simulink library "GTMLE_Library"  (R2014a)
settings: Solver=ode45  StartTime=0.0  StopTime=10.0  RelTol=1e-3
undefined symbols (not defined in the file or in its folder): CCP, DiscIntNeverNeededParam, DPos_test, sample_time, TData_test
undefined symbols (not defined in the file): MCP, steadydata
libraries: simulink x10, GTMLE_Library x2, discretizing x1
(part 2 of 2)

== system GTMLE_Library/Control/Static Control/ /Kp_cor to Kp ==
  Kp_cor : Inport
  T2 : Inport  Port=2
  Fcn : Fcn  Expr=u(1)*sqrt(u(2)/288.15)
  Mux : Mux  Inputs=2
  Kp : Outport
  wires:
  Mux/1 -> Fcn/1
  T2/1 -> Mux/2
  Fcn/1 -> Kp/1
  Kp_cor/1 -> Mux/1

== system GTMLE_Library/Control/Static Control/ /N1_cor ==
  N1 : Inport
  T2 : Inport  Port=2
  Fcn : Fcn  Expr=(u(1)/sqrt(u(2)))*sqrt(288.15)
  Mux : Mux  Inputs=2
  N1cor : Outport
  wires:
  N1/1 -> Mux/1
  Mux/1 -> Fcn/1
  Fcn/1 -> N1cor/1
  T2/1 -> Mux/2

== system GTMLE_Library/Effectors/Iterative NR Solver w JacobianCalc/JC w Reset/Jacobian Calculator ==
  Reset : Inport
  f(x_p) : Inport  Port=2
  Xo : Inport  Port=3
  Constant2 : Constant  Value=N_Per_M
  Counter : Subsystem  mask{N_Ind_M=length(N_Per_M)}
      mask prompts: N_Ind_M "number of independents, N_Ind_M"
  Jacobian : Subsystem
  Terminator : Terminator
  J : Outport
  x_p : Outport  Port=2
  Iteration : Outport  Port=3
  Active : Outport  Port=4
  inv(J) : Outport  Port=5
  wires:
  f(x_p)/1 -> Jacobian/3(f(x_p))
  Constant2/1 -> Jacobian/2(Per)
  Jacobian/1(x_p) -> x_p/1
  Reset/1 -> Counter/1(Reset)
  Counter/1(Enable) -> Active/1, Jacobian/Enable
  Xo/1 -> Jacobian/4(Xo)
  Counter/2(Iteration) -> Iteration/1, Jacobian/1(Iteration)
  Jacobian/2(Inv(J)) -> inv(J)/1
  Jacobian/3(J) -> J/1
  Jacobian/4(y_State) -> Terminator/1

== system GTMLE_Library/Effectors/Iterative NR Solver w JacobianCalc/NRwCond/Iteration Conditions ==
  f(x) : Inport
  Abs : Abs
  Constant1 : Constant  Value=Cond_Limits_M
  Constant2 : Constant  Value=0
  Relational Operator : RelationalOperator  Operator=>  OutDataTypeStr=boolean
  Relational Operator1 : RelationalOperator  Operator=>  OutDataTypeStr=boolean
  Sum of Elements : Sum  Inputs=+
  Condition : Outport
  wires:
  Relational Operator1/1 -> Condition/1
  Sum of Elements/1 -> Relational Operator1/1
  Constant2/1 -> Relational Operator1/2
  Relational Operator/1 -> Sum of Elements/1
  f(x)/1 -> Abs/1
  Constant1/1 -> Relational Operator/2
  Abs/1 -> Relational Operator/1

== system GTMLE_Library/Effectors/Iterative NR Solver w JacobianCalc/NRwCond/Newton Raphson Solver ==
  Enable : Inport
  inv(f'(x(n))) : Inport  Port=2
  f(x(n)) : Inport  Port=3
  Data Type Conversion : DataTypeConversion
  MatrixMult : Subsystem
  Product1 : Product  RndMeth=Zero
  Product2 : Product  RndMeth=Zero
  Sum : Sum  Inputs=|-+
  Unit Delay : UnitDelay  InitialCondition=NR_IC_M  SampleTime=-1
  dxLimit : Subsystem
  x(n+1) : Outport
  y(n) : Outport  Port=2
  wires:
  inv(f'(x(n)))/1 -> Product2/1
  f(x(n))/1 -> Product1/1
  MatrixMult/1(DTS) -> dxLimit/1(dx)
  dxLimit/1(dx_limited) -> Sum/1
  Sum/1 -> y(n)/1, Unit Delay/1
  Unit Delay/1 -> Sum/2, dxLimit/2(dx1), x(n+1)/1
  Product1/1 -> MatrixMult/1(f(x(n)))
  Product2/1 -> MatrixMult/2(inv(f'(x(n))))
  Enable/1 -> Data Type Conversion/1
  Data Type Conversion/1 -> Product1/2, Product2/2

== system GTMLE_Library/Effectors/Iterative NR Solver w JacobianCalc/JC w Reset/Jacobian Calculator/Counter ==
  Reset : Inport
  Constant : Constant
  Constant1 : Constant  Value=N_Ind_M
  Constant2 : Constant  Value=3
  Logical Operator1 : Logic  Operator=NOT  AllPortsSameDT=off  OutDataTypeStr=boolean
  MinMax1 : MinMax  Inputs=2
  Product : Product  RndMeth=Zero
  Relational Operator : RelationalOperator  Operator=>  OutDataTypeStr=boolean
  Sum : Sum  Inputs=|++
  Sum1 : Sum  Inputs=|++
  Unit Delay : UnitDelay  SampleTime=-1
  Enable : Outport
  Iteration : Outport  Port=2
  wires:
  Constant/1 -> Sum/1
  Product/1 -> MinMax1/1
  Sum/1 -> MinMax1/2
  Unit Delay/1 -> Sum/2
  MinMax1/1 -> Unit Delay/1, Iteration/1, Relational Operator/2
  Relational Operator/1 -> Enable/1
  Logical Operator1/1 -> Product/2
  Reset/1 -> Logical Operator1/1
  Sum1/1 -> Relational Operator/1, Product/1
  Constant2/1 -> Sum1/2
  Constant1/1 -> Sum1/1

== system GTMLE_Library/Effectors/Iterative NR Solver w JacobianCalc/JC w Reset/Jacobian Calculator/Jacobian ==
  Iteration : Inport
  Per : Inport  Port=2
  f(x_p) : Inport  Port=3
  Xo : Inport  Port=4
  Enable : EnablePort
  Jacobian Calc : MATLAB Function  TreatAsAtomicUnit=on
  Unit Delay : UnitDelay  InitialCondition=zeros(length(N_Per_M),length(N_Per_M))  SampleTime=-1
  Unit Delay1 : UnitDelay  InitialCondition=zeros(length(N_Per_M),length(N_Per_M)+1)  SampleTime=-1
  Unit Delay2 : UnitDelay  InitialCondition=zeros(length(N_Per_M),1)  SampleTime=-1
  x_p : Outport
  Inv(J) : Outport  Port=2
  J : Outport  Port=3
  y_State : Outport  Port=4
  wires:
  Jacobian Calc/1(XpOut) -> x_p/1
  Xo/1 -> Jacobian Calc/4(XoIn)
  Per/1 -> Jacobian Calc/3(PerIn)
  Iteration/1 -> Jacobian Calc/1(IterationIn)
  Jacobian Calc/3(JOut) -> Unit Delay/1, J/1
  Jacobian Calc/2(InvJOut) -> Inv(J)/1
  Unit Delay/1 -> Jacobian Calc/5(JStateIn)
  Jacobian Calc/4(y_StateOut) -> y_State/1, Unit Delay1/1
  Unit Delay1/1 -> Jacobian Calc/6(y_StateIn)
  f(x_p)/1 -> Unit Delay2/1
  Unit Delay2/1 -> Jacobian Calc/2(y_xpIn)

== system GTMLE_Library/Effectors/Iterative NR Solver w JacobianCalc/NRwCond/Newton Raphson Solver/MatrixMult ==
  f(x(n)) : Inport
  inv(f'(x(n))) : Inport  Port=2
  Product : Product  Multiplication=Matrix(*)  RndMeth=Zero
  DTS : Outport
  wires:
  Product/1 -> DTS/1
  f(x(n))/1 -> Product/2
  inv(f'(x(n)))/1 -> Product/1

== system GTMLE_Library/Effectors/Iterative NR Solver w JacobianCalc/NRwCond/Newton Raphson Solver/dxLimit ==
  dx : Inport
  dx1 : Inport  Port=2
  Abs : Abs
  Constant : Constant  Value=0.5
  Constant1 : Constant  Value=-1
  MinMax : MinMax  Inputs=2
  MinMax1 : MinMax  Function=max  Inputs=2
  Product1 : Product  Inputs=3  RndMeth=Zero
  Product2 : Product  RndMeth=Zero
  Sum : Sum  Inputs=|++
  Threshold : Constant  Value=NR_dx_Lim_M/100
  Unit Delay : UnitDelay  InitialCondition=NR_IC_M  SampleTime=-1
  dx_limited : Outport
  wires:
  MinMax1/1 -> dx_limited/1
  Constant1/1 -> Product2/1
  Product2/1 -> MinMax1/1
  MinMax/1 -> MinMax1/2
  dx/1 -> MinMax/2
  Abs/1 -> Product2/2, MinMax/1
  Product1/1 -> Abs/1
  Threshold/1 -> Product1/1
  dx1/1 -> Sum/2, Unit Delay/1
  Constant/1 -> Product1/2
  Unit Delay/1 -> Sum/1
  Sum/1 -> Product1/3

== matlab function GTMLE_Library/Turbo/Compressor/Comp ==
  data: GasPthCharIn input; GasPthCharOut output; PwrOut output; NErrorOut output; OthrData output; CustBldsCharOut output size=[5 size(CustBldsPlan,2)]; FBldsCharOut output size=[5 size(FBldsPlan,2)]; Nmech input; beta_guess input; VSV input; CustBldsPlan input; FBldsPlan input; Nc_tab input; Beta_tab input; Eff_tab input; PR_tab input; Wc_tab input; SF input; CNST input; WcSurgeVec input; PRSurgeVec input; Msg output
function [ GasPthCharOut, PwrOut, NErrorOut, OthrData, CustBldsCharOut, FBldsCharOut, Msg ] = ComponentsComp( GasPthCharIn, Nmech, beta_guess, VSV, CustBldsPlan, FBldsPlan, Nc_tab, Beta_tab, Eff_tab, PR_tab, Wc_tab, SF, CNST, WcSurgeVec, PRSurgeVec )

[ GasPthCharOut, PwrOut, NErrorOut, OthrData, CustBldsCharOut, FBldsCharOut, Msg ] = Compressor_Untitled( GasPthCharIn, Nmech, beta_guess, VSV, CustBldsPlan, FBldsPlan, Nc_tab, Beta_tab, Eff_tab, PR_tab, Wc_tab, SF, CNST, WcSurgeVec, PRSurgeVec );

end

== matlab function GTMLE_Library/Turbo/Turbine/Turb ==
  data: CoolingFlwCharIn input; GasPthCharIn input size=[5 1]; GasPthCharOut output size=[5 1]; PwrOut output; NErrorOut output; OthrData output; Nmech input; PR input; CoolingPlan input; Nc_tab input; Eff_tab input; PR_tab input; Wc_tab input; SF input; CNST input; Msg output; FuelType input
function [ GasPthCharOut, PwrOut, NErrorOut, OthrData, Msg ] = ComponentsTurb( CoolingFlwCharIn, GasPthCharIn, Nmech, PR, CoolingPlan, Nc_tab, Eff_tab, PR_tab, Wc_tab, SF, CNST, FuelType )

[ GasPthCharOut, PwrOut, NErrorOut, OthrData, Msg ] = Turbine_Untitled( CoolingFlwCharIn, GasPthCharIn, Nmech, PR, CoolingPlan, Nc_tab, Eff_tab, PR_tab, Wc_tab, SF, CNST, FuelType );
   
end

== matlab function GTMLE_Library/Turbo/Duct/Duct ==
  data: GasPthCharIn input size=[5 1]; GasPthCharOut output; CNST input; PtIn_des input; TtIn_des input; WIn_des input; sigma_des input; Blds input; OthrData output
function [ GasPthCharOut, OthrData ]  = ComponentsDuct ( GasPthCharIn , CNST, PtIn_des, TtIn_des, WIn_des, sigma_des, Blds )

[ GasPthCharOut, OthrData ] = Duct_Untitled ( GasPthCharIn , CNST, PtIn_des, TtIn_des, WIn_des, sigma_des, Blds );

end

== matlab function GTMLE_Library/Effectors/Mixer_Ades_calc/MATLAB Function ==
  data: GasPthCharIn1 input; Ades1 output; GasPthCharIn2 input; Mades1 input; Mades2 input; Ades2 output
%%%%%%%%%%%%%%%%%%%%%%%%%%%%%%%%%%
% Untitled -- Mixer_Ades_calc_Untitled.c
% written by Miao Keqiang
% Aeroengine Control Library, Beihang University
% July 12th, 2015

% version 1.0

%%%%%%%%%%%%%%%%%%%%%%%%%%%%%%%%%%

function [ Ades1, Ades2 ] = Mixer_Ades_cal( GasPthCharIn1, GasPthCharIn2, Mades1, Mades2 )

% -- Load data --

WIn1 = 0;
TtIn1 = 0;
PtIn1 = 0;
FARcIn1 = 0;
WIn2 = 0;
TtIn2 = 0;
PtIn2 = 0;
FARcIn2 = 0;

if length( GasPthCharIn1 ) == 5
WIn1 = GasPthCharIn1( 1 );
TtIn1 = GasPthCharIn1( 3 );
PtIn1 = GasPthCharIn1( 4 );
FARcIn1 = GasPthCharIn1( 5 );
end

if length( GasPthCharIn2 ) == 5
WIn2 = GasPthCharIn2( 1 );
TtIn2 = GasPthCharIn2( 3 );
PtIn2 = GasPthCharIn2( 4 );
FARcIn2 = GasPthCharIn2( 5 );
end


% --  Calculate Kq & qlambda1 --

RIn1 = gas_constant( FARcIn1 );
CpIn1 = Cp_T( TtIn1, FARcIn1 );
gammaIn1 = CpIn1 / (CpIn1 - RIn1);
Kqlambda1 = sqrt( gammaIn1/RIn1*( (2/(gammaIn1+1))^((gammaIn1+1)/(gammaIn1-1)) ) );
lambda1 = sqrt( (gammaIn1 + 1) / 2 * Mades1^2 / ( 1 + (gammaIn1 - 1) / 2 * Mades1^2));
qlambdaIn1 = ((gammaIn1 + 1) / 2)^(1 / (gammaIn1 - 1)) * lambda1 * ( 1- (gammaIn1 - 1) / (gammaIn1 + 1) * lambda1^2)^(1 / (gammaIn1 - 1));
Ades1 = ( WIn1 * sqrt( TtIn1 ) ) / ( Kqlambda1 * qlambdaIn1 * PtIn1 * 1e3 );

% --  Calculate lambda2 --

RIn2 = gas_constant( FARcIn2 );
CpIn2 = Cp_T( TtIn2, FARcIn2 );
gammaIn2 = CpIn2 / (CpIn2 - RIn2);
Kqlambda2 = sqrt( gammaIn2/RIn2*( (2/(gammaIn2+1))^((gammaIn2+1)/(gammaIn2-1)) ) );
lambda2 = sqrt( (gammaIn2 + 1) / 2 * Mades2^2 / ( 1 + (gammaIn2 - 1) / 2 * Mades2^2));
qlambdaIn2 = ((gammaIn2 + 1) / 2)^(1 / (gammaIn2 - 1)) * lambda2 * ( 1- (gammaIn2 - 1) / (gammaIn2 + 1) * lambda2^2)^(1 / (gammaIn2 - 1));
Ades2 = ( WIn2 * sqrt( TtIn2 ) ) / ( Kqlambda2 * qlambdaIn2 * PtIn2 * 1e3 );

end

== matlab function GTMLE_Library/Effectors/Iterative NR Solver w JacobianCalc/JC w Reset/Jacobian Calculator/Jacobian/Jacobian Calc ==
  data: IterationIn input; XpOut output; y_xpIn input; PerIn input; XoIn input; InvJOut output; JOut output; JStateIn input; y_StateIn input; y_StateOut output
function [XpOut, InvJOut, JOut, y_StateOut] = fcn(IterationIn, y_xpIn, PerIn, XoIn, JStateIn, y_StateIn)

% Set inital condiations
i = IterationIn;
XpOut = XoIn';
InvJOut = zeros(length(XoIn));
JOut = JStateIn;
y_StateOut = y_StateIn;
% Begin taking data from f(x) at iteration a+1
a = 1;
% Begin determining Jacobian at iteration b+1
b = a+1;

% Set Xp Output
if i > a && i <= length(XoIn) + a
    XpOut(i-a) = XpOut(i-a) + PerIn(i - a);
end

% setup state feedback
if length(XoIn) == 1
    if i == b;
        y_StateOut(1) = y_xpIn;
    end
else
    if i > a && i<= length(XoIn) + a+1;
        y_StateOut(:,i - a) = y_xpIn;
    end
end
% Create Jacobian
if i > b && i <= length(XoIn) + b
    if length(XoIn) == 1
        JOut = (y_xpIn - y_StateIn(1))/PerIn(1);
    else
        JOut(:,i - b) = (y_xpIn - y_StateOut(:,1))/PerIn(i - b);
    end
    if i == length(XoIn) + b
        if rank(JOut) == length(InvJOut)
            InvJOut = inv(JOut(:,:));
        else
%             error('Jacobian can not be inverted.');
        end
    end
end

== matlab function GTMLE_Library/Turbo/Ambient/MATLAB Function1 ==
  data: T1 output; Ma input; P1 output; TH input; PH input; V output
function [T1,P1,V] = fcn(Ma,TH, PH)

     ka = 1.4;
     P1 = PH*(1+((ka-1)/2)*Ma^2)^(ka/(ka-1));
     T1 = TH*(1+((ka-1)/2)*Ma^2);
     
     RSTD = gas_constant( 0 );
     V = Ma * sqrt( ka * RSTD * TH );

end

== matlab function GTMLE_Library/Effectors/LoadTestData/MATLAB Function4 ==
  data: clock input; value output; value_tab input; position_tab input
function value = LoadTestData( clock, value_tab, position_tab )

n = length( position_tab );
value = zeros( 1, n );

for i = 1 : n 
    value( 1, i ) = interp1( value_tab( :, 1 ), value_tab( :, position_tab( i ) ), clock, 'nearest' );
end

end

== matlab function GTMLE_Library/Turbo/Ambient/MATLAB Function2 ==
  data: H input; TH output; PH output; dTs input
function [TH,PH] = fcn(H, dTs)

     P11=2.26e+4;
    
     if H<=11000 
        TH=288.15-6.5*H/1000 + dTs;
        PH=101325*((1-H/44300)^5.255);
     else
        TH=216.5 + dTs;
        PH=P11*exp((11.000-H/1000)/6.318);
     end
     
end

== matlab function GTMLE_Library/Effectors/DesignTools/AccDesign ==
  data: SM input; T4 input; P3 input; n1 output; n2 output; error input; wf_out output; stop output; clock input; n2dot input; SMres input; T4res input; n2_tab input; n2_Wfmin input; kci input; accordec input; statedata input
function [n1,n2,wf_out,stop] = DesignTool(SM, T4, P3, error,clock,n2dot, SMres, T4res, n2_tab, n2_Wfmin, kci, accordec, statedata )

persistent wf;
persistent boss;
if isempty( boss )
    boss = 1;
    wf = statedata( boss, 1 );
end

if ( clock == 0 )
    if ( accordec == 1 )
        fid = fopen( 'AccPlanofWfP3.txt', 'w' );
        fprintf( fid, '********************************\nn2 Wf P3\nrpm kg/s kPa\n' );
        fid = fopen( 'AccPlanofN2dot.txt', 'w' );
        fprintf( fid, '********************************\nn2 n2dot\nrpm rpm/s\n' );
    else
        fid = fopen( 'DecPlanofWfP3.txt', 'w' );
        fprintf( fid, '********************************\nn2 Wf P3\nrpm kg/s kPa\n' );
        fid = fopen( 'DecPlanofN2dot.txt', 'w' );
        fprintf( fid, '********************************\nn2 n2dot\nrpm rpm/s\n' );
    end
    fclose(fid);
end

 n1 = statedata( boss, 2 );
 n2 = statedata( boss, 3 );
 Wfmin = interp1( n2_tab, n2_Wfmin, n2 );
 stop = 0;
 
if ( norm( error, inf ) < kci )
    if ( accordec == 1 )
        if ( SM < SMres || T4 > T4res )
            fid = fopen( 'AccPlanofWfP3.txt', 'a' );
            fprintf( fid, '%g %g %g\n', statedata( boss, 3 ), wf, P3 );
            fid = fopen( 'AccPlanofN2dot.txt', 'a' );
            fprintf( fid, '%g %g\n', statedata(boss,3), n2dot );
            if (  boss < length( statedata )  )
                boss = boss + 1;
            else
                stop = 1;
            end
            wf = statedata( boss, 1 );
            fclose(fid);
        else
            detWF = statedata( boss, 1 ) * 0.01;
            wf = wf + detWF;
        end
    else
        if ( wf < Wfmin )
            fid = fopen( 'DecPlanofWfP3.txt', 'a' );
            fprintf( fid, '%g %g %g\n', statedata( boss, 3 ), wf, P3 );
            fid = fopen( 'DecPlanofN2dot.txt', 'a' );
            fprintf( fid, '%g %g\n', statedata(boss,3), n2dot );
            if (  boss < length( statedata )  )
                boss = boss + 1;
            else
                stop = 1;
            end
            wf = statedata( boss, 1 );
            fclose(fid);
        else
            detWF = statedata( boss, 1 ) * 0.01;
            wf = wf - detWF;
        end
    end
end

wf_out = wf;

== matlab function GTMLE_Library/Turbo/Burner/Burner ==
  data: GasPthCharIn input; GasPthCharOut output; CNST input; dpbur input; LHV input; Eff_des input; PtIn_des input; TtIn_des input; WIn_des input; TtIn_fuel input; Wfin input; FuelType input; Load_tab input; Eff_tab input; SF input; FixEff input; Volume input; OthrData output
function [ GasPthCharOut, OthrData ] = Burner_Untitled ( GasPthCharIn , CNST, dpbur, LHV, Eff_des, PtIn_des, TtIn_des, WIn_des, TtIn_fuel, Wfin, FuelType, Load_tab, Eff_tab, SF, FixEff, Volume )

[ GasPthCharOut, OthrData ] = Burner_Untitled ( GasPthCharIn , CNST, dpbur, LHV, Eff_des, PtIn_des, TtIn_des, WIn_des, TtIn_fuel, Wfin, FuelType, Load_tab, Eff_tab, SF, FixEff, Volume );

end

== matlab function GTMLE_Library/Turbo/Nozzle/Nozzle ==
  data: GasPthCharIn input; WOut output; PambIn input; AthroatIn input; Cdth input; CV input; CX input; FgOut output; NErrorOut output; OthrData output; Msg output
function [ WOut, FgOut, NErrorOut, OthrData, Msg ] = ComponentsNozzle( GasPthCharIn, PambIn, AthroatIn, Cdth, CV, CX )

[ WOut, FgOut, NErrorOut, OthrData, Msg ] = Nozzle_Untitled( GasPthCharIn, PambIn, AthroatIn, Cdth, CV, CX );

end

== matlab function GTMLE_Library/Effectors/SStool/Wf_Schedule ==
  data: Wf_init input; Out_Wf output; Wf_plan input; X input; Err input; Active input; cnt input; stop_flag output; Out_cnt output
function [ Out_Wf, stop_flag, Out_cnt ] = Wf_Schedule( Wf_init, Wf_plan, X, Err, Active, cnt )

stop_flag = 0;
Out_cnt = cnt;
coder.extrinsic('fopen');
coder.extrinsic('fprintf');
coder.extrinsic('fclose');
if ( Active && ~Err )
    
    fid = fopen( 'resource/SS_Tool_Result.txt', 'a' );
    for i = 1 : length( X )
        fprintf( fid, '%f ', X( i ) );
    end
    fprintf( fid, '%f\n', Wf_init * Wf_plan( Out_cnt + 1 ) );
    fclose( fid );
    
    if ( cnt + 1 == length( Wf_plan ) )
        stop_flag = 1;
    else
        Out_cnt = cnt + 1;
    end
end

Out_Wf = Wf_init * Wf_plan( Out_cnt + 1 ); 

end

== matlab function GTMLE_Library/Turbo/Heat Soakage/MATLAB Function ==
  data: TtIn input; Cp output; FARcIn input
function Cp = Cp_T( TtIn, FARcIn )

Cp = Cp_T( TtIn, FARcIn );

== matlab function GTMLE_Library/Turbo/Mixer/Mixer ==
  data: GasPthCharInp input; GasPthCharOut output; Error output; GasPthCharIns input; OthrData output; Adesign1 input; Adesign2 input; Msg output
function [ GasPthCharOut, Error, OthrData, Msg ] = ComponentsMixer( GasPthCharInp, GasPthCharIns, Adesign1, Adesign2 )

[ GasPthCharOut, Error, OthrData, Msg ] = Mixer_Untitled( GasPthCharInp, GasPthCharIns, Adesign1, Adesign2 );

end

== matlab function GTMLE_Library/Control/Acc N1dot/PI1/N1_cor/N1_cor ==
  data: N1 input; N1cor output; T2 input
function N1cor = N1_cor(N1,T2)
N1cor=(N1/sqrt(T2))*sqrt(288.15);
end

== matlab function GTMLE_Library/Control/anti_windup/MinFcn ==
  data: steady input; acc input; choose output; flag output; dec input; acc_N2dot input; flag2 output; dec_N2dot input; flag3 output
function [choose,flag,flag2,flag3] = Min( steady, acc, dec,acc_N2dot,dec_N2dot )
if ( acc < steady )||( acc_N2dot < steady )
    if(acc<=acc_N2dot)
        flag = 1;%冻结稳态控制器积分
        flag2 = 0; %冻结加速ndot控制器积分
        choose = acc;
    else
        flag=1;
        flag2 = 1;
        choose=acc_N2dot;
    end
    flag3 = 0;%冻结减速ndot控制器积分
else
    flag = 0;
    flag2 = 0;
    flag3 = 0;
    choose = steady;
end

if ( dec > choose )||( dec_N2dot > choose )
    if dec >= dec_N2dot
        choose = dec; 
        flag3 = 0;%冻结减速ndot控制器积分
    else
        choose = dec_N2dot; 
        flag3 = 1;
    end
    flag = 1;%冻结稳态控制器积分
	flag2 = 0; %冻结加速ndot控制器积分
end

end
